simulink model "BOOST_design2"  (R2020b)
settings: Solver=ode23tb  StartTime=0.0  StopTime=0.01  MaxStep=1e-6  RelTol=1e-3
libraries: powerlib x11
settings Model: Creator=91845  LastModifiedBy=91845

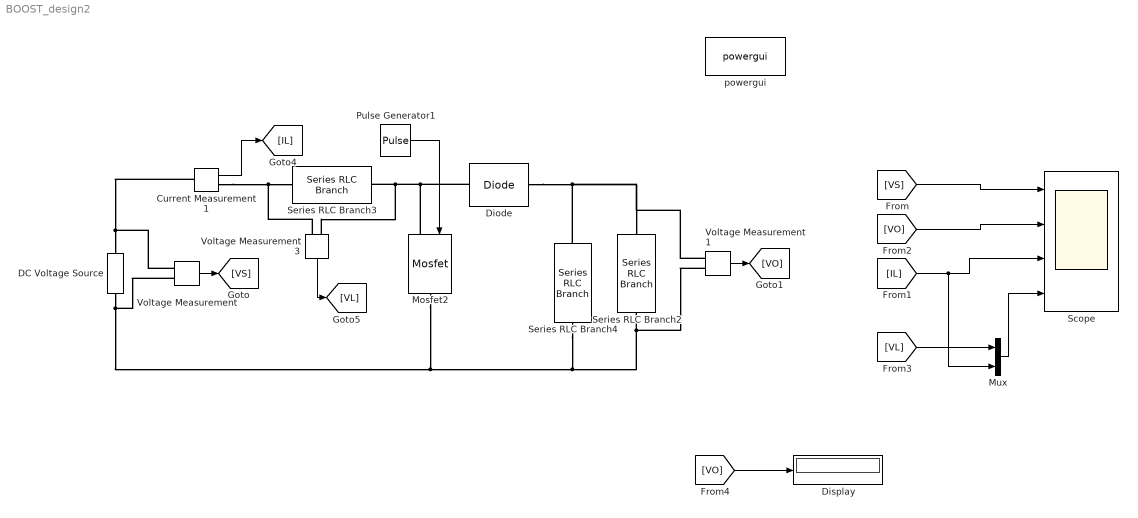
== system BOOST_design2 ==
  Current Measurement1 : powerlib/Measurements/Current Measurement  PhasorSimulation=off  OutputType=Complex  PSBequivalent=0
  DC Voltage Source : powerlib/Electrical Sources/DC Voltage Source  Amplitude=4.2  Measurements=None
  Diode : powerlib/Power Electronics/Diode  Ron=0  Lon=0  Vf=0  IC=0  UseSnubber=0  Rs=inf  Cs=0  Measurements=off
  Display : Display
  Mosfet2 : powerlib/Power Electronics/Mosfet  Ron=0  Lon=0  Rd=0  Vfd=0  IC=0  Rs=1e5  Cs=inf  Measurements=off
  Mux : Mux  Inputs=2
  Pulse Generator1 : DiscretePulseGenerator  PulseType=Time based  Period=(1/200e3)  PulseWidth=0.475*100
  Scope : Scope  NumInputPorts=4
  Series RLC Branch2 : powerlib/Elements/Series RLC Branch  LConnTagsString=__new0  RConnTagsString=__new0  BranchType=R  Resistance=8  Inductance=400e-6  SetiL0=off  InitialCurrent=0  Capacitance=1e-6  Setx0=off  InitialVoltage=0  Measurements=None
  Series RLC Branch3 : powerlib/Elements/Series RLC Branch  LConnTagsString=__new0  RConnTagsString=__new0  BranchType=L  Resistance=1  Inductance=13.1e-6  SetiL0=off  InitialCurrent=0  Capacitance=1e-6  Setx0=off  InitialVoltage=0  Measurements=None
  Series RLC Branch4 : powerlib/Elements/Series RLC Branch  LConnTagsString=__new0  RConnTagsString=__new0  BranchType=RC  Resistance=0.048  Inductance=400e-6  SetiL0=off  InitialCurrent=0  Capacitance=20.7e-6  Setx0=off  InitialVoltage=0  Measurements=Branch voltage
  Voltage Measurement : powerlib/Measurements/Voltage Measurement  PhasorSimulation=off  OutputType=Complex  PSBequivalent=0
  Voltage Measurement1 : powerlib/Measurements/Voltage Measurement  PhasorSimulation=off  OutputType=Complex  PSBequivalent=0
  Voltage Measurement3 : powerlib/Measurements/Voltage Measurement  PhasorSimulation=off  OutputType=Complex  PSBequivalent=0
  powergui : powerlib/powergui  Priority=1  SimulationMode=Continuous  SampleTime=50e-6  frequency=60  Iterations=50  frequencyindice=0  Pbase=100e6  ErrMax=1e-4  UnitsV=kV  UnitsW=MW  buscounter=0  FunctionMessages=off  echomessages=off  EnableUseOfTLC=off  CurrentSourceSwitches=off  DisableSnubberDevices=off  DisableRonSwitches=off  DisableVfSwitches=off  DisplayEquations=off  AutomaticDiscreteSolvers=off  SolverType=Tustin/Backward Euler (TBE)  Interpol=off  ExternalGateDelay=off  methode=off  Ts=100  x0status=blocks  SPID=on  SwTol=0  HookPort=off  NonlinearTolerance=1e-4  nMaxIteration=100  ContinueOnMaxIteration=off  RestoreLinks=warning  ResistiveCurrentMeasurement=off  Frange=[0:2:500]  Ylog=off  Xlog=on  ShowGrid=off  save=off  variable=ZData  structure=0  ZoomFFT=off  StartTime=0.0  cycles=1  DisplayStyle=1  fundamental=60  FreqAxis=off  MaxFrequency=1000  frequencyindicesteady=1  RmsSteady=1  display=off
  wires:
  Voltage Measurement/1 -> [VS]
  Voltage Measurement1/1 -> [VO]
  [VS] -> Scope/1
  [IL] -> Mux/2, Scope/3
  Mux/1 -> Scope/4
  [VO] -> Scope/2
  [VO] -> Display/1
  [VL] -> Mux/1
  Pulse Generator1/1 -> Mosfet2/1
  Voltage Measurement3/1 -> [VL]
  Current Measurement1/1 -> [IL]
  connections:
  Voltage Measurement/LConn1 -- Current Measurement1/LConn1 -- DC Voltage Source/RConn1
  Voltage Measurement1/LConn1 -- Series RLC Branch2/LConn1 -- Series RLC Branch4/RConn1 -- Diode/RConn1
  DC Voltage Source/LConn1 -- Voltage Measurement/LConn2 -- Series RLC Branch4/LConn1 -- Voltage Measurement1/LConn2 -- Series RLC Branch2/RConn1 -- Mosfet2/RConn1
  Current Measurement1/RConn1 -- Series RLC Branch3/LConn1 -- Voltage Measurement3/LConn2
  Diode/LConn1 -- Mosfet2/LConn1 -- Voltage Measurement3/LConn1 -- Series RLC Branch3/RConn1
